simulink model "quadcop_simulator"  (R2020a)
settings: Solver=VariableStepAuto  StartTime=0.0  StopTime=20  RelTol=1e-3
model workspace (MAT data in the model file):
  A = [0  0  0  1  0  0  0  0  0  0  0  0; 0  0  0  0  1  0  0  0  0  0  0  0; 0  0  0  0  0  1  0  0  0  0  0  0; 0  0  0  0  0  0  0  9.81  0  0  0  0; 0  0  0  0  0  0  -9.81  0  0  0  0  0; 0  0  0  0  0  0  0  0  0  0  0  0; 0  0  0  0  0  0  0  0  0  1  0  0; 0  0  0  0  0  0  0  0  0  0  1  0; 0  0  0  0  0  0  0  0  0  0  0  1; 0  0  0  0  0  0  0  0  0  0  0  0; 0  0  0  0  0  0  0  0  0  0  0  0; 0  0  0  0  0  0  0  0  0  0  0  0]
  B = [0  0  0  0; 0  0  0  0; 0  0  0  0; 0  0  0  0; 0  0  0  0; 37.037037037  0  0  0; 0  0  0  0; 0  0  0  0; 0  0  0  0; 0  60551.0873716  -2874.77601308  -1313.13007806; 0  -2874.77601308  60562.1164038  -3654.88622001; 0  -1313.13007806  -3654.88622001  34433.5013278]
  J = [1.657e-05  8.3e-07  7.2e-07; 8.3e-07  1.666e-05  1.8e-06; 7.2e-07  1.8e-06  2.926e-05]
  J2 = [1.657e-05  8.3e-07  7.2e-07; 8.3e-07  1.666e-05  1.8e-06; 7.2e-07  1.8e-06  2.926e-05]
  Jinv = [60551.0873716  -2874.77601308  -1313.13007806; -2874.77601308  60562.1164038  -3654.88622001; -1313.13007806  -3654.88622001  34433.5013278]
  LQR_K = [0  0  0.488031173392  0  0  0.275573390038  0  0  0; 0  -6.19646079613  0  0  -3.23585159473  0  8.09847399024  0  0; 6.19646079613  0  0  3.23585159472  0  0  0  8.09847399024  0; 0  0  0  0  0  0  0  0  1.40922240118]
  M = [1  1  1  1; -0.0325269119346  -0.0325269119346  0.0325269119346  0.0325269119346; -0.0325269119346  0.0325269119346  0.0325269119346  -0.0325269119346; -0.00596  0.00596  -0.00596  0.00596]
  Minv = [0.25  -7.68594327377  -7.68594327377  -41.9463087248; 0.25  -7.68594327377  7.68594327377  41.9463087248; 0.25  7.68594327377  7.68594327377  -41.9463087248; 0.25  7.68594327377  -7.68594327377  41.9463087248]
  NON_LIN_SIM = 1
  T_inner = 0.002
  T_outer = 0.005
  c1 = 6.487e-06
  c2 = 1.3385e-10
  cmd_max = 65535
  cmd_min = 0
  g = 9.81
  m = 0.027
  maxthrust = 0.1597
  nrotor_vehicle_thrust_max = [0.1597; 0.1597; 0.1597; 0.1597]
  pid_x_body_rate_integrator_limit = 33.3
  pid_x_body_rate_ki = 500
  pid_x_body_rate_kp = 250
  pid_y_body_rate_integrator_limit = 33.3
  pid_y_body_rate_ki = 500
  pid_y_body_rate_kp = 250
  pid_z_body_rate_integrator_limit = 167.7
  pid_z_body_rate_ki = 16.7
  pid_z_body_rate_kp = 120
undefined symbols (not defined in the file or in its folder): measurement_noise_full_state_covariance_decomposition, measurement_noise_full_state_mean, measurement_noise_full_state_seed, measurement_noise_gyroscope_covariance_decomposition, measurement_noise_gyroscope_mean, measurement_noise_gyroscope_seed, measurement_noise_gyroscope_var, sample_time_measurements_body_rates, sample_time_measurements_full_state, sigbuilder_block
libraries: vrlib x1
settings Model: OrderedModelArguments=off  Creator=Ben  LastModifiedBy=Ben

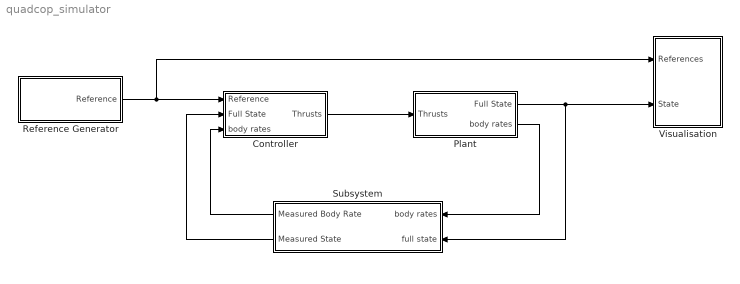
== system quadcop_simulator ==
  Controller : Subsystem
  Plant : Subsystem
  Reference Generator : Subsystem
  Subsystem : Subsystem
  Visualisation : Subsystem
  wires:
  Reference Generator/1(Reference) -> Visualisation/1(References), Controller/1(Reference)
  Controller/1(Thrusts) -> Plant/1(Thrusts)
  Plant/1(Full State) -> Subsystem/2(full state), Visualisation/2(State)
  Subsystem/2(Measured State) -> Controller/2(Full State)
  Subsystem/1(Measured Body Rate) -> Controller/3(body rates)
  Plant/2(body rates) -> Subsystem/1(body rates)

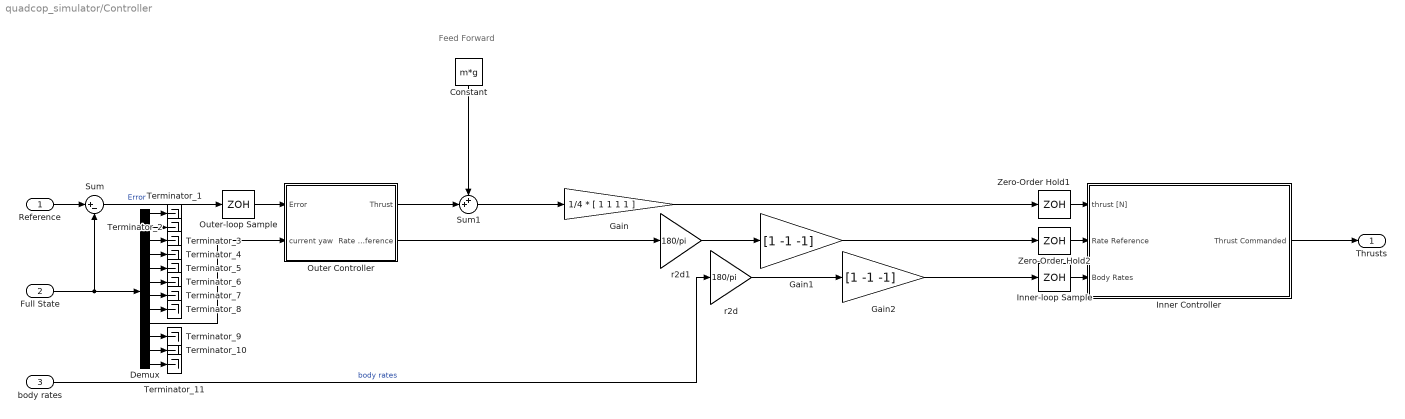
== system quadcop_simulator/Controller ==
  note: Feed Forward
  Reference : Inport  PortDimensions=12
  Full State : Inport  Port=2  PortDimensions=12
  body rates : Inport  Port=3
  Constant : Constant  Value=m*g
  Demux : Demux  Outputs=12
  Gain : Gain  Gain=1/4 * [ 1 1 1 1 ]
  Gain1 : Gain  Gain=[1 -1 -1]
  Gain2 : Gain  Gain=[1 -1 -1]
  Inner Controller : Subsystem
  Inner-loop Sample : ZeroOrderHold  SampleTime=T_inner
  Outer Controller : Subsystem
  Outer-loop Sample : ZeroOrderHold  SampleTime=T_outer
  Sum : Sum  Inputs=|+-
  Sum1 : Sum  Inputs=++|
  Terminator_{1..11} (11 alike) : Terminator
  Zero-Order Hold1 : ZeroOrderHold  SampleTime=T_inner
  Zero-Order Hold2 : ZeroOrderHold  SampleTime=T_inner
  r2d : Gain  Gain=180/pi
  r2d1 : Gain  Gain=180/pi
  Thrusts : Outport
  wires:
  Constant/1 -> Sum1/1
  Reference/1 -> Sum/1
  Full State/1 -> Sum/2, Demux/1
  Sum/1 -> Outer-loop Sample/1  "Error"
  Outer Controller/2(Rate Reference) -> r2d1/1
  Outer Controller/1(Thrust) -> Sum1/2
  Inner-loop Sample/1 -> Inner Controller/3(Body Rates)
  Zero-Order Hold2/1 -> Inner Controller/2(Rate Reference)
  Zero-Order Hold1/1 -> Inner Controller/1(thrust [N])
  Outer-loop Sample/1 -> Outer Controller/1(Error)
  Gain/1 -> Zero-Order Hold1/1
  Sum1/1 -> Gain/1
  Inner Controller/1(Thrust Commanded) -> Thrusts/1
  body rates/1 -> r2d/1  "body rates"
  r2d/1 -> Gain2/1
  r2d1/1 -> Gain1/1
  Gain1/1 -> Zero-Order Hold2/1
  Gain2/1 -> Inner-loop Sample/1
  Demux/9 -> Outer Controller/2(current yaw)
  Demux/1 -> Terminator_1/1
  Demux/2 -> Terminator_2/1
  Demux/3 -> Terminator_3/1
  Demux/4 -> Terminator_4/1
  Demux/5 -> Terminator_5/1
  Demux/6 -> Terminator_6/1
  Demux/7 -> Terminator_7/1
  Demux/8 -> Terminator_8/1
  Demux/10 -> Terminator_9/1
  Demux/11 -> Terminator_10/1
  Demux/12 -> Terminator_11/1

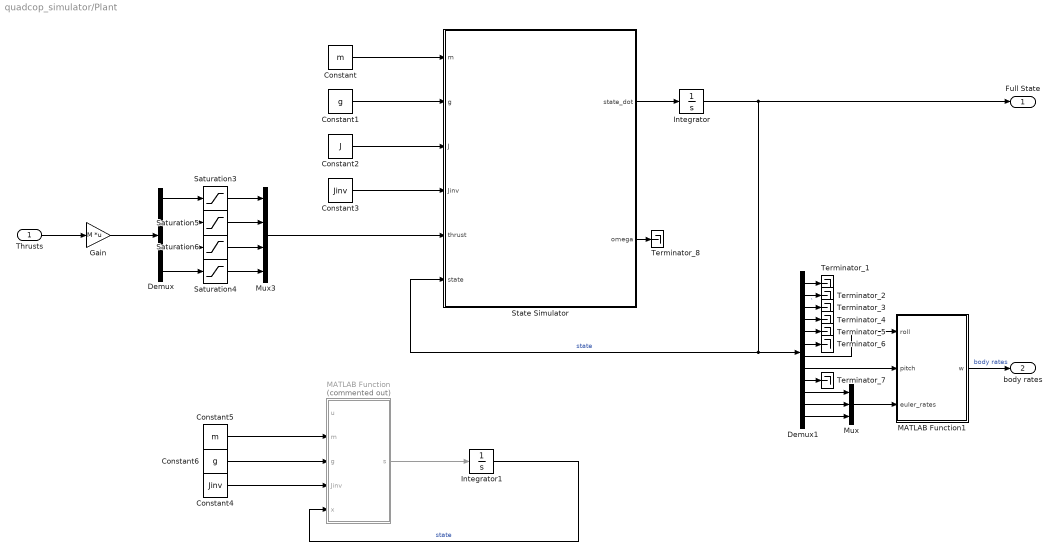
== system quadcop_simulator/Plant ==
  Thrusts : Inport  PortDimensions=[4 1]
  Constant : Constant  Value=m
  Constant1 : Constant  Value=g
  Constant2 : Constant  Value=J
  Constant3 : Constant  Value=Jinv
  Constant4 : Constant  Value=Jinv
  Constant5 : Constant  Value=m
  Constant6 : Constant  Value=g
  Demux : Demux
  Demux1 : Demux  Outputs=12
  Gain : Gain  Gain=M  Multiplication=Matrix(K*u)
  Integrator : Integrator
  Integrator1 : Integrator
  MATLAB Function : MATLAB Function  Commented=on  TreatAsAtomicUnit=on
  MATLAB Function1 : MATLAB Function  TreatAsAtomicUnit=on
  Mux : Mux  Inputs=3
  Mux3 : Mux
  Saturation3 : Saturate  UpperLimit=4*maxthrust  LowerLimit=0
  Saturation4 : Saturate  UpperLimit=0.0119*maxthrust  LowerLimit=-0.0119*maxthrust
  Saturation5 : Saturate  UpperLimit=0.0651*maxthrust  LowerLimit=-0.0651*maxthrust
  Saturation6 : Saturate  UpperLimit=0.0651*maxthrust  LowerLimit=-0.0651*maxthrust
  State Simulator : MATLAB Function  TreatAsAtomicUnit=on
  Terminator_{1..8} (8 alike) : Terminator
  Full State : Outport  PortDimensions=12
  body rates : Outport  Port=2
  wires:
  State Simulator/1(state_dot) -> Integrator/1
  Integrator/1 -> Full State/1, Demux1/1, State Simulator/6(state)  "state"
  Constant/1 -> State Simulator/1(m)
  Constant1/1 -> State Simulator/2(g)
  Constant3/1 -> State Simulator/4(Jinv)
  Constant2/1 -> State Simulator/3(J)
  Thrusts/1 -> Gain/1
  Integrator1/1 -> MATLAB Function/5(x)  "state"
  MATLAB Function/1(s) -> Integrator1/1
  Constant5/1 -> MATLAB Function/2(m)
  Constant6/1 -> MATLAB Function/3(g)
  Constant4/1 -> MATLAB Function/4(Jinv)
  Saturation5/1 -> Mux3/2
  Demux/3 -> Saturation6/1
  Saturation3/1 -> Mux3/1
  Demux/1 -> Saturation3/1
  Mux3/1 -> State Simulator/5(thrust)
  Demux/2 -> Saturation5/1
  Demux/4 -> Saturation4/1
  Saturation4/1 -> Mux3/4
  Gain/1 -> Demux/1
  Saturation6/1 -> Mux3/3
  Demux1/10 -> Mux/1
  Demux1/11 -> Mux/2
  Demux1/12 -> Mux/3
  Mux/1 -> MATLAB Function1/3(euler_rates)
  Demux1/7 -> MATLAB Function1/1(roll)
  Demux1/8 -> MATLAB Function1/2(pitch)
  MATLAB Function1/1(w) -> body rates/1  "body rates"
  Demux1/1 -> Terminator_1/1
  Demux1/2 -> Terminator_2/1
  Demux1/3 -> Terminator_3/1  "`"
  Demux1/4 -> Terminator_4/1
  Demux1/5 -> Terminator_5/1
  Demux1/6 -> Terminator_6/1
  Demux1/9 -> Terminator_7/1
  State Simulator/2(omega) -> Terminator_8/1

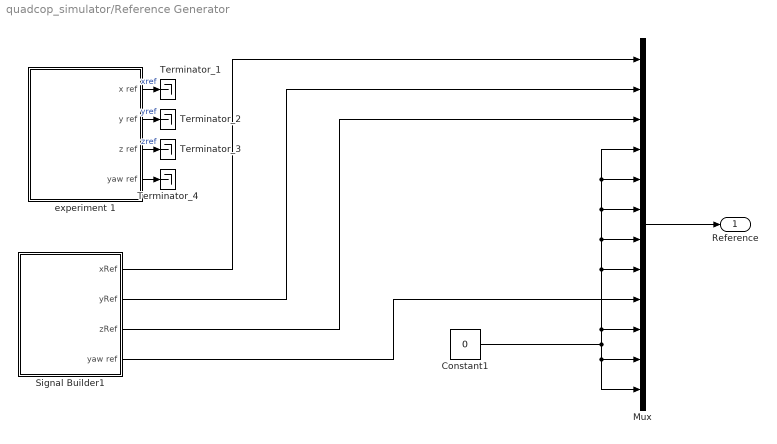
== system quadcop_simulator/Reference Generator ==
  Constant1 : Constant  Value=0
  Mux : Mux  Inputs=12
  Signal Builder1 : Subsystem  Tag=STV Subsys  LoadFcn=sigbuilder_block('load');  StartFcn=sigbuilder_block('start');  StopFcn=sigbuilder_block('stop');  ClipboardFcn=sigbuilder_block('clipboard');  mask(Sigbuilder block){tuvar=[0:10]}
      mask help: Simulink:masks:SigbuilderBlock_MD
      mask init:
      | if ~strcmp(get_param(bdroot(gcbh),'SimulationStatus'),'stopped') tuvar = sigbuilder_block('maskInit'); end
      settings: CopyFcn=sigbuilder_block('copy');  DeleteFcn=sigbuilder_block('delete');  ModelCloseFcn=sigbuilder_block('modelClose');  PreSaveFcn=sigbuilder_block('preSave');  PauseFcn=sigbuilder_block('pause');  ContinueFcn=sigbuilder_block('continue');  NameChangeFcn=sigbuilder_block('namechange');  OpenFcn=sigbuilder_block('open',[255.375 171.75 864.75 431.625 ]);  CloseFcn=sigbuilder_block('close');
      mask Display: plot(0, 0, 100, 100,[2, 2, 32, 32, 2], [68, 8, 8, 68, 68],[32, 2], [38, 38], [32, 19, 2],[53, 60, 44], [32, 17, 17, 2],[16, 16, 31, 31]);txt = getActiveGroup(gcbh);text(2, 100, txt,'verticalAlignment', 'top');
  Terminator_{1..4} (4 alike) : Terminator
  experiment 1 : Subsystem  Tag=STV Subsys  LoadFcn=sigbuilder_block('load');  StartFcn=sigbuilder_block('start');  StopFcn=sigbuilder_block('stop');  ClipboardFcn=sigbuilder_block('clipboard');  mask(Sigbuilder block){tuvar=[0:10]}
      mask help: Simulink:masks:SigbuilderBlock_MD
      mask init:
      | if ~strcmp(get_param(bdroot(gcbh),'SimulationStatus'),'stopped') tuvar = sigbuilder_block('maskInit'); end
      settings: CopyFcn=sigbuilder_block('copy');  DeleteFcn=sigbuilder_block('delete');  ModelCloseFcn=sigbuilder_block('modelClose');  PreSaveFcn=sigbuilder_block('preSave');  PauseFcn=sigbuilder_block('pause');  ContinueFcn=sigbuilder_block('continue');  NameChangeFcn=sigbuilder_block('namechange');  OpenFcn=sigbuilder_block('open',[4.875 30 1115.25 631.875 ]);  CloseFcn=sigbuilder_block('close');
      mask Display: plot(0, 0, 100, 100,[2, 2, 32, 32, 2], [68, 8, 8, 68, 68],[32, 2], [38, 38], [32, 19, 2],[53, 60, 44], [32, 17, 17, 2],[16, 16, 31, 31]);txt = getActiveGroup(gcbh);text(2, 100, txt,'verticalAlignment', 'top');
  Reference : Outport
  wires:
  Mux/1 -> Reference/1
  Constant1/1 -> Mux/12, Mux/11, Mux/5, Mux/4, Mux/6, Mux/7, Mux/8, Mux/10
  Signal Builder1/1(xRef) -> Mux/1
  Signal Builder1/2(yRef) -> Mux/2
  Signal Builder1/3(zRef) -> Mux/3
  Signal Builder1/4(yaw ref) -> Mux/9
  experiment 1/1(x ref) -> Terminator_1/1  "xref"
  experiment 1/2(y ref) -> Terminator_2/1  "yref"
  experiment 1/3(z ref) -> Terminator_3/1  "zref"
  experiment 1/4(yaw ref) -> Terminator_4/1

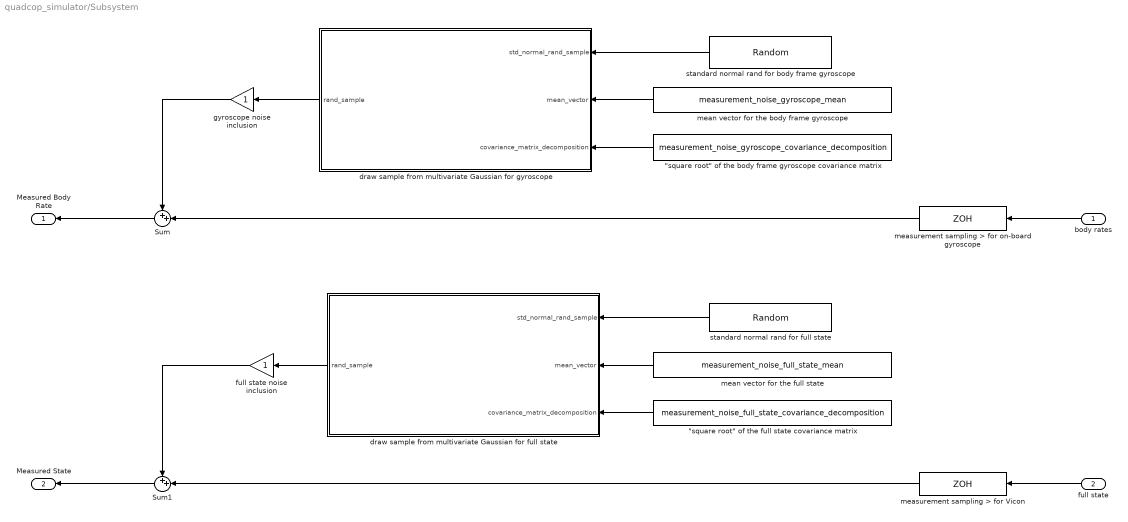
== system quadcop_simulator/Subsystem ==
  body rates : Inport
  full state : Inport  Port=2
  "\"square root\" of the body frame gyroscope covariance matrix" : Constant  Value=measurement_noise_gyroscope_covariance_decomposition
  "\"square root\" of the full state covariance matrix" : Constant  Value=measurement_noise_full_state_covariance_decomposition
  Sum : Sum  Inputs=++|
  Sum1 : Sum  Inputs=++|
  draw sample from multivariate Gaussian for full state : MATLAB Function  TreatAsAtomicUnit=on
  draw sample from multivariate Gaussian for gyroscope : MATLAB Function  TreatAsAtomicUnit=on
  full state noise inclusion : Gain
  gyroscope noise inclusion : Gain
  mean vector for the body frame gyroscope : Constant  Value=measurement_noise_gyroscope_mean
  mean vector for the full state : Constant  Value=measurement_noise_full_state_mean
  measurement sampling > for Vicon : ZeroOrderHold  SampleTime=sample_time_measurements_full_state
  measurement sampling > for on-board gyroscope : ZeroOrderHold  SampleTime=sample_time_measurements_body_rates
  standard normal rand for body frame gyroscope : RandomNumber  Mean=measurement_noise_gyroscope_mean  Variance=measurement_noise_gyroscope_var  Seed=measurement_noise_gyroscope_seed  SampleTime=sample_time_measurements_body_rates  VectorParams1D=off
  standard normal rand for full state : RandomNumber  Mean=zeros(12,1)  Variance=ones(12,1)  Seed=measurement_noise_full_state_seed  SampleTime=sample_time_measurements_full_state  VectorParams1D=off
  Measured Body Rate : Outport
  Measured State : Outport  Port=2
  wires:
  Sum1/1 -> Measured State/1
  Sum/1 -> Measured Body Rate/1
  "\"square root\" of the full state covariance matrix"/1 -> draw sample from multivariate Gaussian for full state/3(covariance_matrix_decomposition)
  full state noise inclusion/1 -> Sum1/1
  mean vector for the full state/1 -> draw sample from multivariate Gaussian for full state/2(mean_vector)
  mean vector for the body frame gyroscope/1 -> draw sample from multivariate Gaussian for gyroscope/2(mean_vector)
  measurement sampling > for on-board gyroscope/1 -> Sum/2
  standard normal rand for full state/1 -> draw sample from multivariate Gaussian for full state/1(std_normal_rand_sample)
  "\"square root\" of the body frame gyroscope covariance matrix"/1 -> draw sample from multivariate Gaussian for gyroscope/3(covariance_matrix_decomposition)
  standard normal rand for body frame gyroscope/1 -> draw sample from multivariate Gaussian for gyroscope/1(std_normal_rand_sample)
  full state/1 -> measurement sampling > for Vicon/1
  draw sample from multivariate Gaussian for gyroscope/1(rand_sample) -> gyroscope noise inclusion/1
  draw sample from multivariate Gaussian for full state/1(rand_sample) -> full state noise inclusion/1
  body rates/1 -> measurement sampling > for on-board gyroscope/1
  measurement sampling > for Vicon/1 -> Sum1/2
  gyroscope noise inclusion/1 -> Sum/1

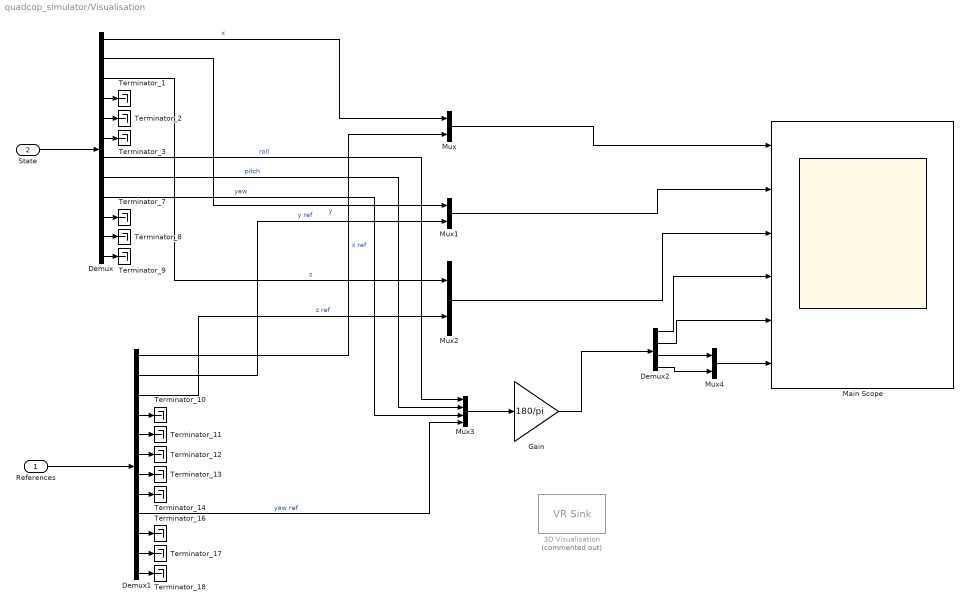
== system quadcop_simulator/Visualisation ==
  References : Inport
  State : Inport  Port=2
  3D Visualisation : vrlib/VR Sink  Commented=on  InstantiateOnLoad=on  SampleTime=0.1  ViewEnable=on  RemoteChange=off  RemoteView=off  WorldFileName=asbQuadcopterAHBase.wrl  AutoView=off  VideoDimensions=[]  AllowVariableSize=off
  Demux : Demux  Outputs=12
  Demux1 : Demux  Outputs=12
  Demux2 : Demux
  Gain : Gain  Gain=180/pi
  Main Scope : Scope  NumInputPorts=6
  Mux{,1..2,4} (4 alike) : Mux  Inputs=2
  Mux3 : Mux
  Terminator_{1..3,7..14,16..18} (14 alike) : Terminator
  wires:
  References/1 -> Demux1/1
  State/1 -> Demux/1
  Demux/1 -> Mux/1  "x"
  Demux1/1 -> Mux/2  "x ref"
  Mux/1 -> Main Scope/1
  Demux/2 -> Mux1/1  "y"
  Demux1/2 -> Mux1/2  "y ref"
  Demux1/3 -> Mux2/2  "z ref"
  Demux/3 -> Mux2/1  "z"
  Mux1/1 -> Main Scope/2
  Mux2/1 -> Main Scope/3
  Demux/4 -> Terminator_1/1
  Demux/5 -> Terminator_2/1
  Demux/6 -> Terminator_3/1
  Demux/7 -> Mux3/1  "roll"
  Demux/8 -> Mux3/2  "pitch"
  Demux/9 -> Mux3/3  "yaw"
  Demux/10 -> Terminator_7/1
  Demux/11 -> Terminator_8/1
  Demux/12 -> Terminator_9/1
  Demux1/4 -> Terminator_10/1
  Demux1/5 -> Terminator_11/1
  Demux1/6 -> Terminator_12/1
  Demux1/7 -> Terminator_13/1
  Demux1/8 -> Terminator_14/1
  Demux1/9 -> Mux3/4  "yaw ref"
  Demux1/10 -> Terminator_16/1
  Demux1/11 -> Terminator_17/1
  Demux1/12 -> Terminator_18/1
  Mux3/1 -> Gain/1
  Gain/1 -> Demux2/1
  Demux2/3 -> Mux4/1
  Demux2/4 -> Mux4/2
  Mux4/1 -> Main Scope/6
  Demux2/2 -> Main Scope/5
  Demux2/1 -> Main Scope/4

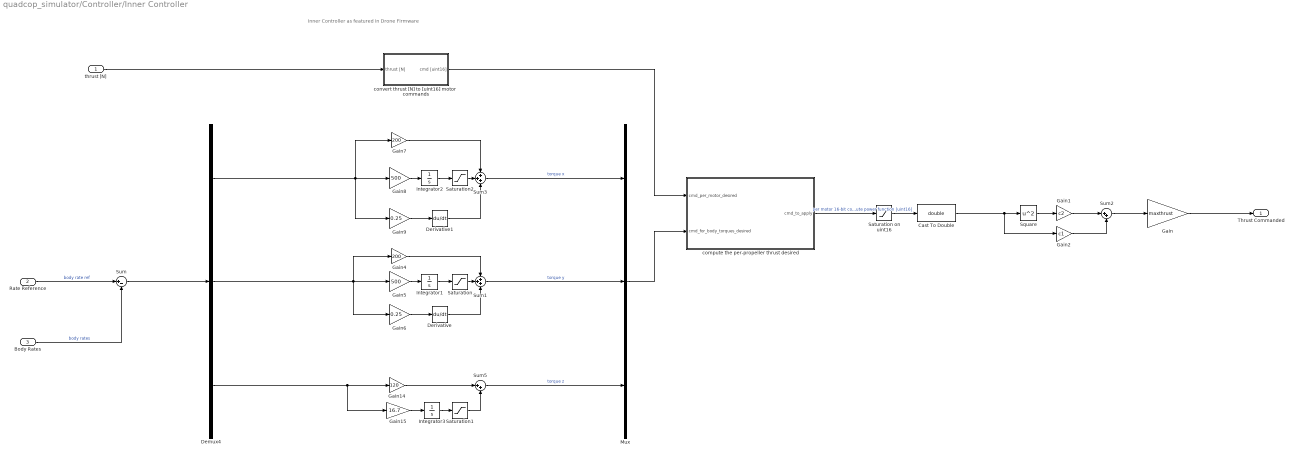
== system quadcop_simulator/Controller/Inner Controller ==
  note: Inner Controller as featured in Drone Firmware
  thrust [N] : Inport  PortDimensions=4
  Rate Reference : Inport  Port=2  PortDimensions=3
  Body Rates : Inport  Port=3  PortDimensions=3
  Cast To Double : DataTypeConversion  OutDataTypeStr=double
  Demux4 : Demux  Outputs=3
  Derivative : Derivative
  Derivative1 : Derivative
  Gain : Gain  Gain=maxthrust
  Gain1 : Gain  Gain=c2
  Gain14 : Gain  Gain=120
  Gain15 : Gain  Gain=16.7
  Gain2 : Gain  Gain=c1
  Gain4 : Gain  Gain=200
  Gain5 : Gain  Gain=500
  Gain6 : Gain  Gain=0.25
  Gain7 : Gain  Gain=200
  Gain8 : Gain  Gain=500
  Gain9 : Gain  Gain=0.25
  Integrator1 : Integrator
  Integrator2 : Integrator
  Integrator3 : Integrator
  Mux : Mux  Inputs=3
  Saturation : Saturate  UpperLimit=33.3  LowerLimit=-33.3
  Saturation on uint16 : Saturate  UpperLimit=cmd_max  LowerLimit=cmd_min  ZeroCross=off
  Saturation1 : Saturate  UpperLimit=167.7  LowerLimit=-167.7
  Saturation2 : Saturate  UpperLimit=33.3  LowerLimit=-33.3
  Square : Math  Operator=square  SignedPower=on  SaturateOnIntegerOverflow=on
  Sum : Sum  Inputs=|+-
  Sum1 : Sum  Inputs=+++
  Sum2 : Sum  Inputs=|++
  Sum3 : Sum  Inputs=+++
  Sum5 : Sum  Inputs=|++
  compute the per-propeller thrust desired : MATLAB Function  TreatAsAtomicUnit=on
  convert thrust [N] to [uint16] motor commands : Subsystem
  Thrust Commanded : Outport  PortDimensions=[4 1]
  wires:
  Mux/1 -> compute the per-propeller thrust desired/2(cmd_for_body_torques_desired)
  compute the per-propeller thrust desired/1(cmd_to_apply) -> Saturation on uint16/1  "per motor 16-bit command after distribute power function [uint16]"
  Rate Reference/1 -> Sum/1  "body rate ref"
  convert thrust [N] to [uint16] motor commands/1(cmd [uint16]) -> compute the per-propeller thrust desired/1(cmd_per_motor_desired)
  thrust [N]/1 -> convert thrust [N] to [uint16] motor commands/1(thrust [N])
  Gain2/1 -> Sum2/2
  Gain1/1 -> Sum2/1
  Cast To Double/1 -> Gain2/1, Square/1
  Square/1 -> Gain1/1
  Saturation on uint16/1 -> Cast To Double/1
  Body Rates/1 -> Sum/2  "body rates"
  Integrator1/1 -> Saturation/1
  Gain4/1 -> Sum1/1
  Demux4/2 -> Gain6/1, Gain5/1, Gain4/1
  Gain5/1 -> Integrator1/1
  Sum1/1 -> Mux/2  "torque y"
  Gain15/1 -> Integrator3/1
  Sum5/1 -> Mux/3  "torque z"
  Gain14/1 -> Sum5/1
  Integrator3/1 -> Saturation1/1
  Demux4/3 -> Gain15/1, Gain14/1
  Gain6/1 -> Derivative/1
  Derivative/1 -> Sum1/3
  Sum3/1 -> Mux/1  "torque x"
  Demux4/1 -> Gain9/1, Gain8/1, Gain7/1
  Gain8/1 -> Integrator2/1
  Gain9/1 -> Derivative1/1
  Integrator2/1 -> Saturation2/1
  Derivative1/1 -> Sum3/3
  Gain7/1 -> Sum3/1
  Sum/1 -> Demux4/1
  Saturation/1 -> Sum1/2
  Saturation1/1 -> Sum5/2
  Saturation2/1 -> Sum3/2
  Sum2/1 -> Gain/1
  Gain/1 -> Thrust Commanded/1

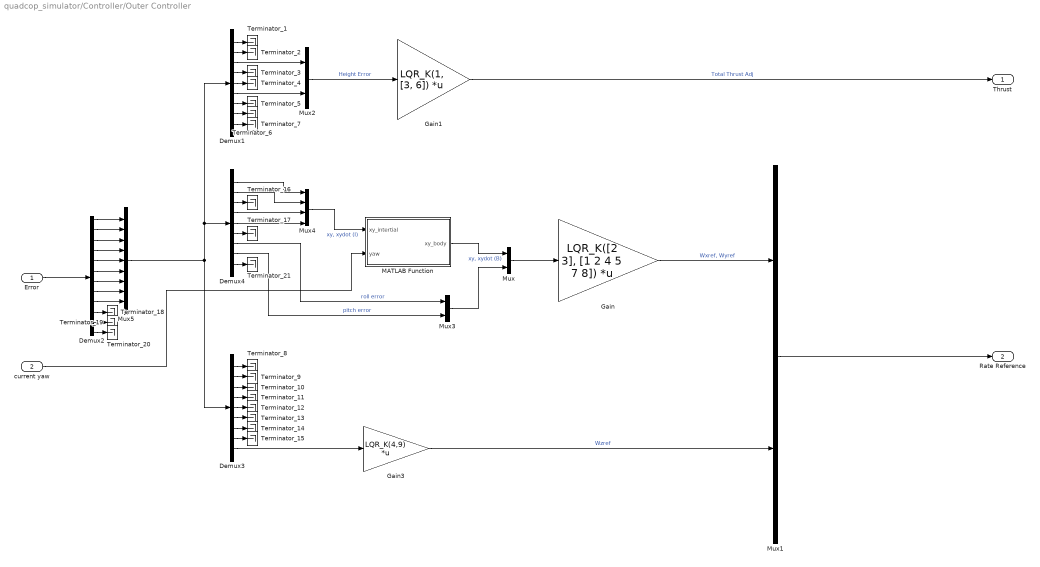
== system quadcop_simulator/Controller/Outer Controller ==
  Error : Inport  PortDimensions=12
  current yaw : Inport  Port=2
  Demux1 : Demux  Outputs=9
  Demux2 : Demux  Outputs=12
  Demux3 : Demux  Outputs=9
  Demux4 : Demux  Outputs=9
  Gain : Gain  Gain=LQR_K([2 3], [1 2 4 5 7 8])  Multiplication=Matrix(K*u)
  Gain1 : Gain  Gain=LQR_K(1, [3, 6])  Multiplication=Matrix(K*u)
  Gain3 : Gain  Gain=LQR_K(4,9)  Multiplication=Matrix(K*u)
  MATLAB Function : MATLAB Function  TreatAsAtomicUnit=on
  Mux{,1..3} (4 alike) : Mux  Inputs=2
  Mux4 : Mux
  Mux5 : Mux  Inputs=9
  Terminator_{1..21} (21 alike) : Terminator
  Thrust : Outport  PortDimensions=[1 1]
  Rate Reference : Outport  Port=2  PortDimensions=3
  wires:
  Mux5/1 -> Demux4/1, Demux1/1, Demux3/1
  Mux2/1 -> Gain1/1  "Height Error"
  Gain3/1 -> Mux1/2  "Wzref"
  Mux1/1 -> Rate Reference/1
  Mux4/1 -> MATLAB Function/1(xy_intertial)  "xy, xydot (I)"
  MATLAB Function/1(xy_body) -> Mux/1  "xy, xydot (B)"
  Mux/1 -> Gain/1
  Gain/1 -> Mux1/1  "Wxref, Wyref"
  Demux1/3 -> Mux2/1
  Demux1/6 -> Mux2/2
  Error/1 -> Demux2/1
  Demux3/9 -> Gain3/1
  Demux4/1 -> Mux4/1
  Demux4/2 -> Mux4/2
  Demux4/4 -> Mux4/3
  Demux4/5 -> Mux4/4
  Demux4/7 -> Mux3/1  "roll error"
  Demux4/8 -> Mux3/2  "pitch error"
  Demux2/1 -> Mux5/1
  Demux2/2 -> Mux5/2
  Demux2/3 -> Mux5/3
  Demux2/4 -> Mux5/4
  Demux2/5 -> Mux5/5
  Demux2/6 -> Mux5/6
  Demux2/7 -> Mux5/7
  Demux2/8 -> Mux5/8
  Demux2/9 -> Mux5/9
  Demux1/1 -> Terminator_1/1
  Demux1/2 -> Terminator_2/1
  Demux1/4 -> Terminator_3/1
  Demux1/5 -> Terminator_4/1
  Demux1/7 -> Terminator_5/1
  Demux1/8 -> Terminator_6/1
  Demux1/9 -> Terminator_7/1
  Demux3/1 -> Terminator_8/1
  Demux3/2 -> Terminator_9/1
  Demux3/3 -> Terminator_10/1
  Demux3/4 -> Terminator_11/1
  Demux3/5 -> Terminator_12/1
  Demux3/6 -> Terminator_13/1
  Demux3/7 -> Terminator_14/1
  Demux3/8 -> Terminator_15/1
  Demux4/3 -> Terminator_16/1
  Demux4/6 -> Terminator_17/1
  Demux2/10 -> Terminator_18/1
  Demux2/11 -> Terminator_19/1
  Demux2/12 -> Terminator_20/1
  Gain1/1 -> Thrust/1  "Total Thrust Adj"
  Mux3/1 -> Mux/2
  current yaw/1 -> MATLAB Function/2(yaw)
  Demux4/9 -> Terminator_21/1

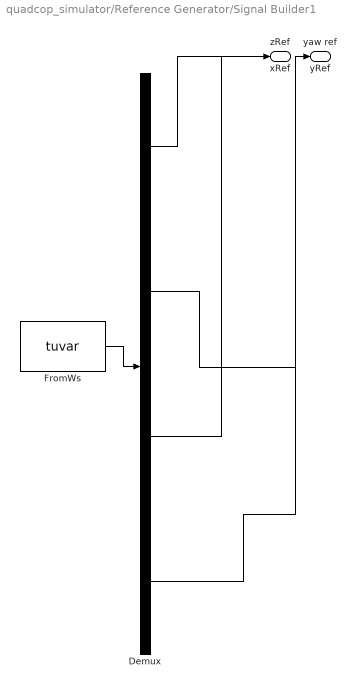
== system quadcop_simulator/Reference Generator/Signal Builder1 ==
  Demux : Demux  Tag=STV Demux
      settings: DisplayOption=none
  FromWs : FromWorkspace  Tag=STV FromWs  VariableName=tuvar
      SigBuilderData=|
      | common.afterFinalStr = 'Extrapolate'
      | common.sampleTime = 0
      | dataSet.timeRange = [0 30]
      | dataSet.name = 'Group 1'
      | sbobj.Groups.Name = 'Group 1'
      | sbobj.Groups.Signals(1).Name = 'xRef'
      | sbobj.Groups.Signals(1).XData = [0 5 5 30]
      | sbobj.Groups.Signals(1).YData = [0 0 1 1]
      | sbobj.Groups.Signals(2).Name = 'yRef'
      | sbobj.Groups.Signals(2).XData = [0 15 15 30]
      | sbobj.Groups.Signals(2).YData = [0 0 1 1]
      | sbobj.Groups.Signals(3).Name = 'zRef'
      | sbobj.Groups.Signals(3).XData = [0 1 1 2 2 30]
      | sbobj.Groups.Signals(3).YData = [0.3 0.3 0.5 0.5 0.7 0.7]
      | sbobj.Groups.Signals(4).Name = 'yaw ref'
      | sbobj.Groups.Signals(4).XData = [0 5.2 5.2 30]
      | sbobj.Groups.Signals(4).YData = [0 0 1 1]
      | sbobj.Groups.TimeRange = [0 30]
  xRef : Outport  Tag=STV Outport
  yRef : Outport  Tag=STV Outport  Port=2
  zRef : Outport  Tag=STV Outport  Port=3
  yaw ref : Outport  Tag=STV Outport  Port=4
  wires:
  FromWs/1 -> Demux/1
  Demux/1 -> xRef/1
  Demux/2 -> yRef/1
  Demux/3 -> zRef/1
  Demux/4 -> yaw ref/1

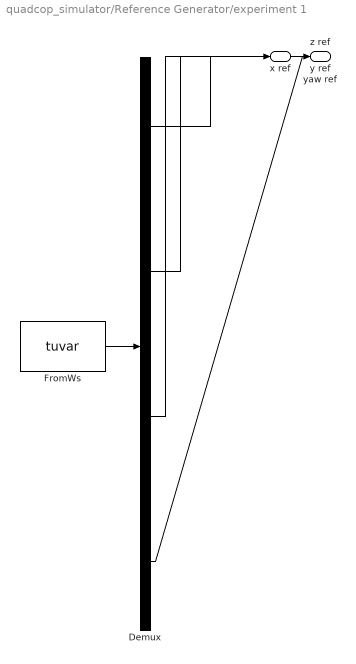
== system quadcop_simulator/Reference Generator/experiment 1 ==
  Demux : Demux  Tag=STV Demux
      settings: DisplayOption=none
  FromWs : FromWorkspace  Tag=STV FromWs  VariableName=tuvar
      SigBuilderData=|
      | common.afterFinalStr = 'Extrapolate'
      | common.sampleTime = 0
      | dataSet.timeRange = [0 10]
      | dataSet.name = 'Group 1'
      | sbobj.Groups.Name = 'Group 1'
      | sbobj.Groups.Signals(1).Name = 'x ref'
      | sbobj.Groups.Signals(1).XData = [0 8 8 10]
      | sbobj.Groups.Signals(1).YData = [0 0 1 1]
      | sbobj.Groups.Signals(2).Name = 'y ref'
      | sbobj.Groups.Signals(2).XData = [0 5 5 10]
      | sbobj.Groups.Signals(2).YData = [0 0 1 1]
      | sbobj.Groups.Signals(3).Name = 'z ref'
      | sbobj.Groups.Signals(3).XData = [0 1 1 10]
      | sbobj.Groups.Signals(3).YData = [0 0 1 1]
      | sbobj.Groups.Signals(4).Name = 'yaw ref'
      | sbobj.Groups.Signals(4).XData = [0 2.01 2.01 10]
      | sbobj.Groups.Signals(4).YData = [0 0 1 1]
  x ref : Outport  Tag=STV Outport
  y ref : Outport  Tag=STV Outport  Port=2
  z ref : Outport  Tag=STV Outport  Port=3
  yaw ref : Outport  Tag=STV Outport  Port=4
  wires:
  Demux/1 -> x ref/1
  FromWs/1 -> Demux/1
  Demux/2 -> y ref/1
  Demux/3 -> z ref/1
  Demux/4 -> yaw ref/1

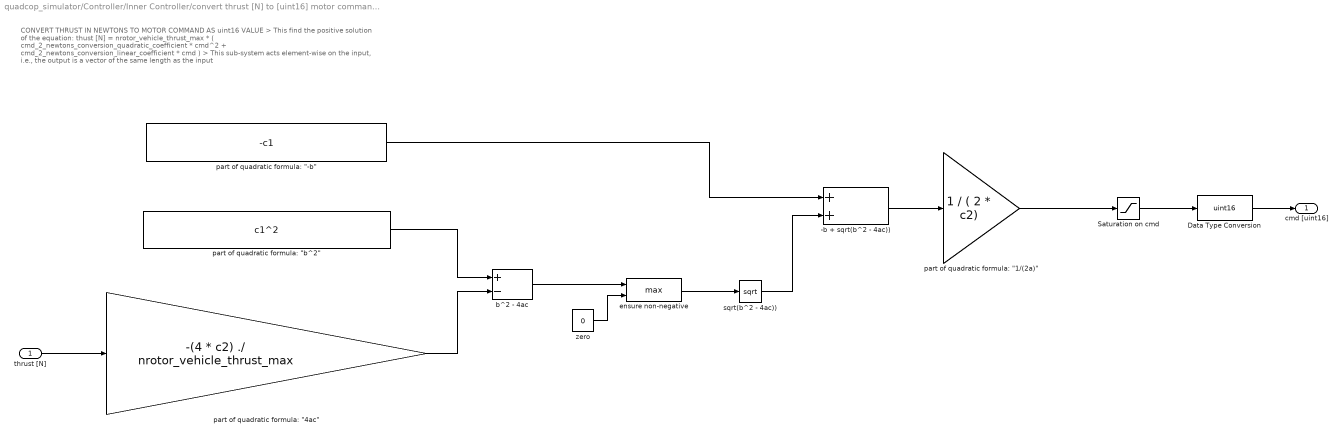
== system quadcop_simulator/Controller/Inner Controller/convert thrust [N] to [uint16] motor commands ==
  note: CONVERT THRUST IN NEWTONS TO MOTOR COMMAND AS uint16 VALUE
      | > This find the positive solution of the equation:
      | thust [N] = nrotor_vehicle_thrust_max * ( cmd_2_newtons_conversion_quadratic_coefficient * cmd^2 + cmd_2_newtons_conversion_linear_coefficient * cmd )
      |
      | > This sub-system acts element-wise on the input, i.e., the output is a vector of the same length as the input
  thrust [N] : Inport
  -b + sqrt(b^2 - 4ac)) : Sum
  Data Type Conversion : DataTypeConversion  OutDataTypeStr=uint16
  Saturation on cmd : Saturate  UpperLimit=cmd_max  LowerLimit=cmd_min  ZeroCross=off
  b^2 - 4ac : Sum  Inputs=+-
  ensure non-negative : MinMax  Function=max  Inputs=2
  "part of quadratic formula: \"-b\"" : Constant  Value=-c1
  "part of quadratic formula: \"1/(2a)\"" : Gain  Gain=1 / ( 2 * c2)
  "part of quadratic formula: \"4ac\"" : Gain  Gain=-(4 * c2) ./ nrotor_vehicle_thrust_max
  "part of quadratic formula: \"b^2\"" : Constant  Value=c1^2
  sqrt(b^2 - 4ac)) : Sqrt  SaturateOnIntegerOverflow=on
  zero : Constant  Value=0
  cmd [uint16] : Outport  VectorParamsAs1DForOutWhenUnconnected=off
  wires:
  thrust [N]/1 -> "part of quadratic formula: \"4ac\""/1
  Saturation on cmd/1 -> Data Type Conversion/1
  Data Type Conversion/1 -> cmd [uint16]/1
  "part of quadratic formula: \"4ac\""/1 -> b^2 - 4ac/2
  "part of quadratic formula: \"b^2\""/1 -> b^2 - 4ac/1
  b^2 - 4ac/1 -> ensure non-negative/1
  ensure non-negative/1 -> sqrt(b^2 - 4ac))/1
  "part of quadratic formula: \"-b\""/1 -> -b + sqrt(b^2 - 4ac))/1
  sqrt(b^2 - 4ac))/1 -> -b + sqrt(b^2 - 4ac))/2
  -b + sqrt(b^2 - 4ac))/1 -> "part of quadratic formula: \"1/(2a)\""/1
  "part of quadratic formula: \"1/(2a)\""/1 -> Saturation on cmd/1
  zero/1 -> ensure non-negative/2

== matlab function quadcop_simulator/Controller/Outer Controller/MATLAB Function ==
  data: xy_intertial input; yaw input; xy_body output
function xy_body = fbRi(xy_intertial, yaw)

    bRi = [ cos(yaw) sin(yaw); -sin(yaw) cos(yaw) ];
    
    xy_body = [ bRi, zeros(2); zeros(2), bRi ] * xy_intertial;

== matlab function quadcop_simulator/Plant/State Simulator ==
  data: m input; g input; J input; Jinv input; thrust input; state_dot output; state input; omega output
function [state_dot, omega] = quad_dynamics(m, g, J, Jinv, thrust,state)

ftotal = thrust(1);


pos_dot = state(4:6);
euler = state(7:9);
euler_dot = state(10:12);

roll = euler(1);
pitch = euler(2);
yaw = euler(3);
roll_dot = euler_dot(1);
pitch_dot = euler_dot(2);
% yaw_dot = euler_dot(3);

% roll, pitch, yaw

iRb = [ cos(pitch)*cos(yaw),   -cos(roll)*sin(yaw) + sin(roll)*sin(pitch)*cos(yaw),    sin(roll)*sin(yaw) + cos(roll)*sin(pitch)*cos(yaw);
        cos(pitch)*sin(yaw),   cos(roll)*cos(yaw) + sin(roll)*sin(pitch)*sin(yaw),     -sin(roll)*cos(yaw) + cos(roll)*sin(pitch)*sin(yaw);
        -sin(pitch),           cos(pitch)*sin(roll),                                   cos(pitch)*cos(roll)];

T = [ 1,    0,          -sin(pitch);
      0,    cos(roll),   sin(roll)*cos(pitch);
      0,    -sin(roll),  cos(roll)*cos(pitch)];

Tinv = [    1,     sin(roll)*tan(pitch),    cos(roll)*tan(pitch);
            0,     cos(roll),               -sin(roll);
            0,     sin(roll)*sec(pitch),    cos(roll)*sec(pitch)];

Tdot = [    0,  0,                      -cos(pitch) * pitch_dot;
            0,  -sin(roll) * roll_dot,    -sin(roll)*sin(pitch)*pitch_dot + cos(roll)*cos(pitch)*roll_dot;
            0   -cos(roll) * roll_dot,    -cos(roll)*sin(pitch)*pitch_dot - sin(roll)*cos(pitch) * roll_dot];

omega = T * euler_dot;
omega_dot = Jinv * ( thrust(2:4) - cross(omega, J*omega) );
euler_dotdot = Tinv * ( omega_dot - Tdot * euler_dot );

pos_dotdot = 1/m * ( iRb * [0; 0; ftotal] - [0; 0; m*g]);

state_dot = [   pos_dot;
                pos_dotdot;
                euler_dot; 
                euler_dotdot ];

== matlab function quadcop_simulator/Plant/MATLAB Function ==
  data: u input; m input; g input; Jinv input; x input; s output
function s = semilinear_plant(u, m, g, Jinv, x)

yaw = x(9);

u(1) = u(1) - m * g;

A = [zeros(12,3), [blkdiag(eye(3), g*[sin(yaw) cos(yaw) 0; -cos(yaw) sin(yaw) 0; 0 0 0], eye(3)); zeros(3,9)]];
B = [ zeros(3,4); zeros(2,4); [1/m zeros(1,3)]; zeros(3,4); [ zeros(3,1), Jinv]];

s = A*x + B*u;

== matlab function quadcop_simulator/Controller/Inner Controller/compute the per-propeller thrust desired ==
  data: cmd_per_motor_desired input; cmd_for_body_torques_desired input; cmd_to_apply output
function cmd_to_apply = distribute_power( cmd_per_motor_desired , cmd_for_body_torques_desired )
% ----------------------------------------------------------------------- %
% DESCRIPTION:
% This function computes the uint16 command to apply to each motor as per
% the code that runs "on-board" on the Crazyflie's firmware
%
%
% INPUT ARGUMENTS:
%
% cmd_per_motor_desired [uint16]
% > This is a colulmn vector with length equal to the number of propellers
%   on the Crazyflie, i.e., 4, and each element represents the "baseline"
%   16-bit command that should be requested from the Crazyflie, as
%   requested by the outer loop controller.
%
% cmd_for_body_torques_desired [uint16]
% > This is the "actuation" uint16 command that comes directly from the
%   output of the Crazyflie's body rate PID controllers running in the
%   firmware. This value of command has already been adjust for the
%   dimensions of the Crazyflie, and the pattern for distributing the
%   command across the motor is provided in the exercise sheet.
%
%
% RETURN ARGUMENTS:
% % cmd_to_apply [uint16]
% > This is a colulmn vector with length equal to the number of propellers
%   on the Crazyflie, i.e., 4, and each element represents the 16-bit
%   command that will be requested from the motors
%
%
% DATA FORMAT ASSUMPTIONS:
% > the "cmd_per_motor_desired" vector is such when applied, the static
%   thrusts exert no torque about the body frame axes
%
% ----------------------------------------------------------------------- %


% Get the uint16 commands into a separate variable for each motor
cmd1 = cmd_per_motor_desired(1);
cmd2 = cmd_per_motor_desired(2);
cmd3 = cmd_per_motor_desired(3);
cmd4 = cmd_per_motor_desired(4);


% Get the desired body torques uint16 commands into a separate variable for
% the "uint16 command torque" desired about each of the body frame axes
r = cmd_for_body_torques_desired(1) / 2;
p = cmd_for_body_torques_desired(2) / 2;
y = cmd_for_body_torques_desired(3);


% These variable names have been used to partially match the code from the
% Crazyflie firmware:
% r  -  where "r" stands for roll, this is the "uint16 command torque" to
%       apply about the body-frame's x-axis, i.e., the roll-axis
% p  -  where "p" stands for pitch, this is the "uint16 command torque" to
%       apply about the body-frame's y-axis, i.e., the pitch-axis
% y  -  where "y" stands for yaw, this is the "uint16 command torque" to
%       apply about the body-frame's z-axis, i.e., the yaw-axis
%
% Note: the "/ 2" for the extraction of "r" and "p" above is simply added
% to minimic the code of the Crazyflie firmware. Presumably the Crazyflie's
% PID contollers for the body-frame roll and pitch axis are tuned with this
% factor of "/ 2" appropriately accounted for.


% Initialise the return variable "cmd_to_apply" to zeros
% > This can be required so that Simulink knows the expected size
cmd_to_apply = zeros(4,1);

% Compute the 16-bit command that should be applied from each motor as per
% the code from the Crazyflie firmware
% > For motor 1:
cmd_to_apply(1,1)  =  cmd1   - r   + p  +  y;
% > For motor 1:
cmd_to_apply(2,1)  =  cmd2   - r   - p  -  y;
% > For motor 1:
cmd_to_apply(3,1)  =  cmd3   + r   - p  +  y;
% > For motor 1:
cmd_to_apply(4,1)  =  cmd4   + r   + p  -  y;

== matlab function quadcop_simulator/Subsystem/draw sample from multivariate Gaussian for full state ==
  data: std_normal_rand_sample input; rand_sample output; mean_vector input; covariance_matrix_decomposition input
function rand_sample = mvn_full_state( std_normal_rand_sample , mean_vector , covariance_matrix_decomposition )


% Compute the multi-variate Gaussian sample from a distirbution with:
% > "mean_vector" as the mean, and
% > "covariance_matrix_decomposition" as the "square root" of the
%    covariance matrix
rand_sample = mean_vector + covariance_matrix_decomposition * std_normal_rand_sample;

== matlab function quadcop_simulator/Subsystem/draw sample from multivariate Gaussian for gyroscope ==
  data: std_normal_rand_sample input; rand_sample output; mean_vector input; covariance_matrix_decomposition input
function rand_sample = mvn_gyroscope( std_normal_rand_sample , mean_vector , covariance_matrix_decomposition )


% Compute the multi-variate Gaussian sample from a distirbution with:
% > "mean_vector" as the mean, and
% > "covariance_matrix_decomposition" as the "square root" of the
%    covariance matrix
rand_sample = mean_vector + covariance_matrix_decomposition * std_normal_rand_sample;

== matlab function quadcop_simulator/Plant/MATLAB Function1 ==
  data: roll input; pitch input; euler_rates input; w output
function w = Trot(roll, pitch, euler_rates)
T = [ 1,    0,          -sin(pitch);
      0,    cos(roll),   sin(roll)*cos(pitch);
      0,    -sin(roll),  cos(roll)*cos(pitch)];
 w = T * euler_rates;
